simulink model "zad1_2"  (R2020a)
settings: Solver=FixedStepDiscrete  StartTime=0.0  StopTime=0.0  RelTol=1e-3
libraries: CPOiS_SourcesSinks x8, CPOiS_LinearTransforms x4, CPOiS_DataManipulation_DataTypeConversion x2
settings Model: Creator=johnb  LastModifiedBy=johnb

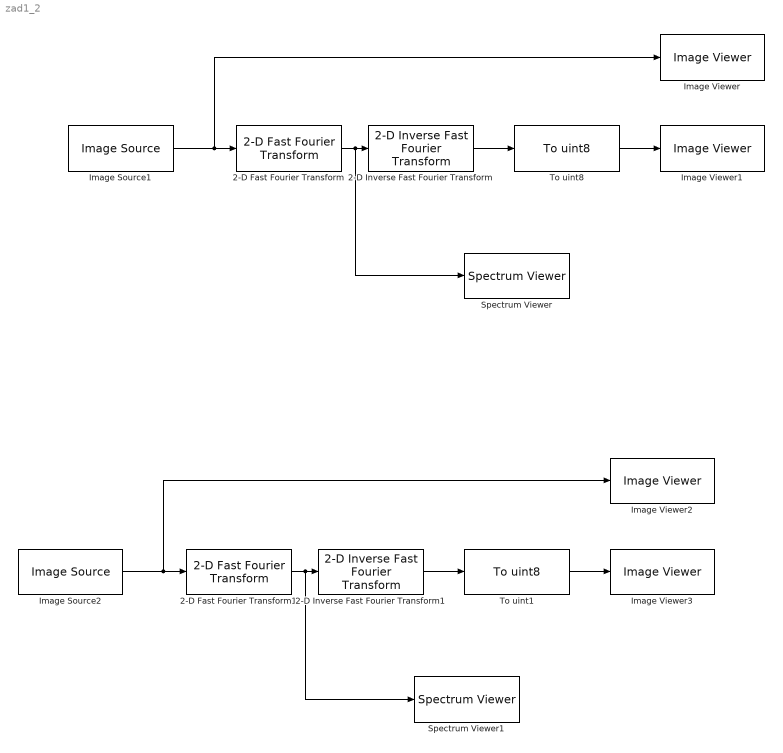
== system zad1_2 ==
  2-D Fast Fourier Transform : CPOiS_LinearTransforms/2-D Fast Fourier Transform
      settings: SourceProductName=CPOiS - Digital image and signal processing
  2-D Fast Fourier Transform1 : CPOiS_LinearTransforms/2-D Fast Fourier Transform
      settings: SourceProductName=CPOiS - Digital image and signal processing
  2-D Inverse Fast Fourier Transform : CPOiS_LinearTransforms/2-D Inverse Fast  Fourier Transform
      settings: SourceProductName=CPOiS - Digital image and signal processing
  2-D Inverse Fast Fourier Transform1 : CPOiS_LinearTransforms/2-D Inverse Fast  Fourier Transform
      settings: SourceProductName=CPOiS - Digital image and signal processing
  Image Source1 : CPOiS_SourcesSinks/Image Source  FileSelection=ball.png
      settings: SourceProductName=CPOiS - Digital image and signal processing
  Image Source2 : CPOiS_SourcesSinks/Image Source  FileSelection=gull.png
      settings: SourceProductName=CPOiS - Digital image and signal processing
  Image Viewer{,1..3} (4 alike) : CPOiS_SourcesSinks/Image Viewer
      settings: SourceProductName=CPOiS - Digital image and signal processing
  Spectrum Viewer : CPOiS_SourcesSinks/Spectrum Viewer
      settings: SourceProductName=CPOiS - Digital image and signal processing
  Spectrum Viewer1 : CPOiS_SourcesSinks/Spectrum Viewer
      settings: SourceProductName=CPOiS - Digital image and signal processing
  To uint1 : CPOiS_DataManipulation_DataTypeConversion/To uint8
      settings: SourceProductName=CPOiS - Digital image and signal processing
  To uint8 : CPOiS_DataManipulation_DataTypeConversion/To uint8
      settings: SourceProductName=CPOiS - Digital image and signal processing
  wires:
  Image Source1/1 -> Image Viewer/1, 2-D Fast Fourier Transform/1
  2-D Fast Fourier Transform/1 -> Spectrum Viewer/1, 2-D Inverse Fast Fourier Transform/1
  2-D Inverse Fast Fourier Transform/1 -> To uint8/1
  To uint8/1 -> Image Viewer1/1
  To uint1/1 -> Image Viewer3/1
  2-D Inverse Fast Fourier Transform1/1 -> To uint1/1
  2-D Fast Fourier Transform1/1 -> Spectrum Viewer1/1, 2-D Inverse Fast Fourier Transform1/1
  Image Source2/1 -> Image Viewer2/1, 2-D Fast Fourier Transform1/1
